simulink library "accs"  (Simulink 8.1)
settings: Solver=ode45  StartTime=0.0  StopTime=10.0  RelTol=1e-3
undefined symbols (not defined in the file or in its folder): ENUM_ACCSTATE_OFF, ENUM_ACCSTATE_STANDBY
settings Model: Creator=AT015555  LastModifiedBy=tescamilla

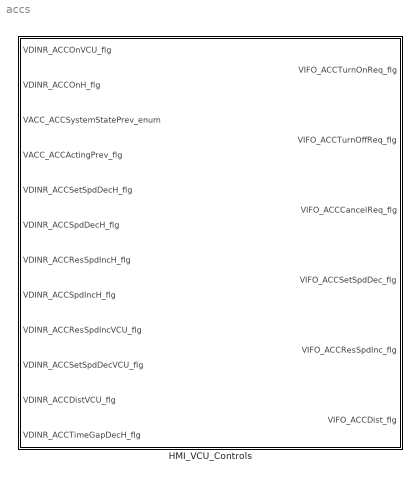
== system accs ==
  HMI_VCU_Controls : Subsystem

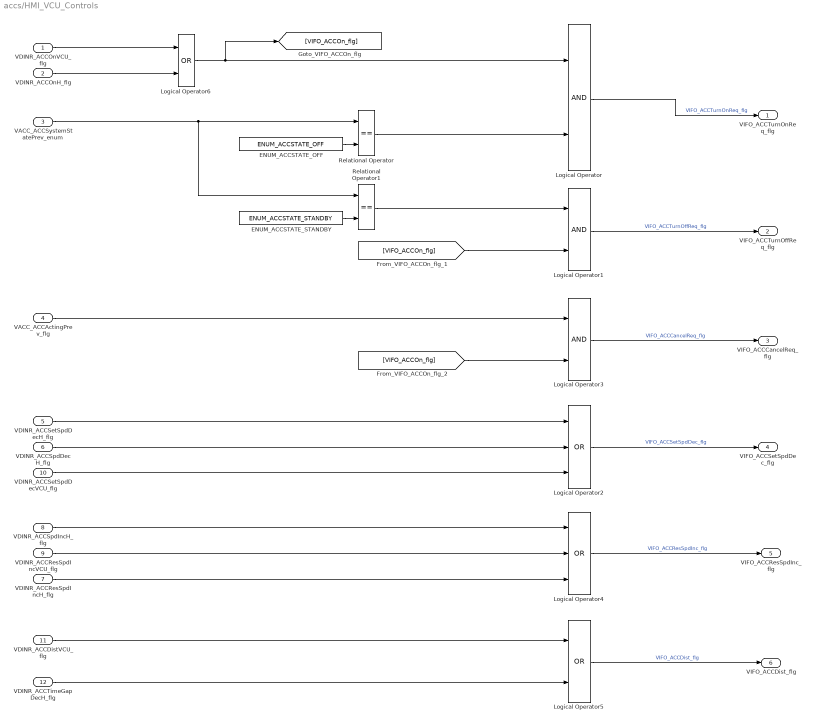
== system accs/HMI_VCU_Controls ==
  VDINR_ACCOnVCU_flg : Inport
  VDINR_ACCOnH_flg : Inport  Port=2
  VACC_ACCSystemStatePrev_enum : Inport  Port=3
  VACC_ACCActingPrev_flg : Inport  Port=4
  VDINR_ACCSetSpdDecH_flg : Inport  Port=5
  VDINR_ACCSpdDecH_flg : Inport  Port=6
  VDINR_ACCResSpdIncH_flg : Inport  Port=7
  VDINR_ACCSpdIncH_flg : Inport  Port=8
  VDINR_ACCResSpdIncVCU_flg : Inport  Port=9
  VDINR_ACCSetSpdDecVCU_flg : Inport  Port=10
  VDINR_ACCDistVCU_flg : Inport  Port=11
  VDINR_ACCTimeGapDecH_flg : Inport  Port=12
  ENUM_ACCSTATE_OFF : Constant  Value=ENUM_ACCSTATE_OFF
  ENUM_ACCSTATE_STANDBY : Constant  Value=ENUM_ACCSTATE_STANDBY
  Logical Operator : Logic  AllPortsSameDT=off  OutDataTypeStr=boolean
  Logical Operator1 : Logic  AllPortsSameDT=off  OutDataTypeStr=boolean
  Logical Operator2 : Logic  Operator=OR  Inputs=3  AllPortsSameDT=off  OutDataTypeStr=boolean
  Logical Operator3 : Logic  AllPortsSameDT=off  OutDataTypeStr=boolean
  Logical Operator4 : Logic  Operator=OR  Inputs=3  AllPortsSameDT=off  OutDataTypeStr=boolean
  Logical Operator5 : Logic  Operator=OR  AllPortsSameDT=off  OutDataTypeStr=boolean
  Logical Operator6 : Logic  Operator=OR  AllPortsSameDT=off  OutDataTypeStr=boolean
  Relational Operator : RelationalOperator  Operator===  OutDataTypeStr=boolean
  Relational Operator1 : RelationalOperator  Operator===  OutDataTypeStr=boolean
  VIFO_ACCTurnOnReq_flg : Outport
  VIFO_ACCTurnOffReq_flg : Outport  Port=2
  VIFO_ACCCancelReq_flg : Outport  Port=3
  VIFO_ACCSetSpdDec_flg : Outport  Port=4
  VIFO_ACCResSpdInc_flg : Outport  Port=5
  VIFO_ACCDist_flg : Outport  Port=6
  wires:
  Relational Operator/1 -> Logical Operator/2
  ENUM_ACCSTATE_OFF/1 -> Relational Operator/2
  ENUM_ACCSTATE_STANDBY/1 -> Relational Operator1/2
  VDINR_ACCOnVCU_flg/1 -> Logical Operator6/1
  Logical Operator6/1 -> Logical Operator/1, [VIFO_ACCOn_flg]
  [VIFO_ACCOn_flg] -> Logical Operator1/2
  Relational Operator1/1 -> Logical Operator1/1
  Logical Operator/1 -> VIFO_ACCTurnOnReq_flg/1  "VIFO_ACCTurnOnReq_flg"
  Logical Operator1/1 -> VIFO_ACCTurnOffReq_flg/1  "VIFO_ACCTurnOffReq_flg"
  VACC_ACCSystemStatePrev_enum/1 -> Relational Operator/1, Relational Operator1/1
  [VIFO_ACCOn_flg] -> Logical Operator3/2
  Logical Operator3/1 -> VIFO_ACCCancelReq_flg/1  "VIFO_ACCCancelReq_flg"
  VACC_ACCActingPrev_flg/1 -> Logical Operator3/1
  VDINR_ACCSetSpdDecVCU_flg/1 -> Logical Operator2/3
  VDINR_ACCSetSpdDecH_flg/1 -> Logical Operator2/1
  VDINR_ACCSpdDecH_flg/1 -> Logical Operator2/2
  VDINR_ACCResSpdIncVCU_flg/1 -> Logical Operator4/2
  VDINR_ACCSpdIncH_flg/1 -> Logical Operator4/1
  VDINR_ACCResSpdIncH_flg/1 -> Logical Operator4/3
  Logical Operator2/1 -> VIFO_ACCSetSpdDec_flg/1  "VIFO_ACCSetSpdDec_flg"
  VDINR_ACCTimeGapDecH_flg/1 -> Logical Operator5/2
  VDINR_ACCDistVCU_flg/1 -> Logical Operator5/1
  Logical Operator4/1 -> VIFO_ACCResSpdInc_flg/1  "VIFO_ACCResSpdInc_flg"
  Logical Operator5/1 -> VIFO_ACCDist_flg/1  "VIFO_ACCDist_flg"
  VDINR_ACCOnH_flg/1 -> Logical Operator6/2
